simulink library "Library"  (R2017b)
settings: Solver=ode45  StartTime=0.0  StopTime=10.0  RelTol=1e-3  EnableMultiTasking=on
libraries: simulink x1
settings Model: Creator=Administrator  LastModifiedBy=ZhuDeShui
settings DataIOCC: LimitDataPoints=on  SaveFormat=Array
settings OptimizationCC: LifeSpan=inf
settings DebuggingCC: SolverPrmCheckMsg=warning  AllowSymbolicDim=off  SFUnexpectedBacktrackingDiag=warning  SFNoUnconditionalDefaultTransitionDiag=warning  SFExecutionAtInitializationDiag=none
settings HardwareCC: ProdBitPerPointer=32  ProdBitPerSizeT=32  ProdBitPerPtrDiffT=32  ProdLargestAtomicFloat=None  ProdIntDivRoundTo=Undefined  ProdEndianess=Unspecified  ProdWordSize=32  ProdHWDeviceType=32-bit Generic
settings ModelReferenceCC: PropagateSignalLabelsOutOfModel=off
settings CodeAppCC: StateflowObjectComments=on
settings GRTTargetCC: TargetLangStandard=C89/C90 (ANSI)  GeneratePreprocessorConditionals=Disable all
settings ConfigComp: CovMetricSettings=dw  CovHtmlReporting=on  CovSaveCumulativeToWorkspaceVar=on  CovSaveSingleToWorkspaceVar=on  CovExternalEMLEnable=off  CovSFcnEnable=off

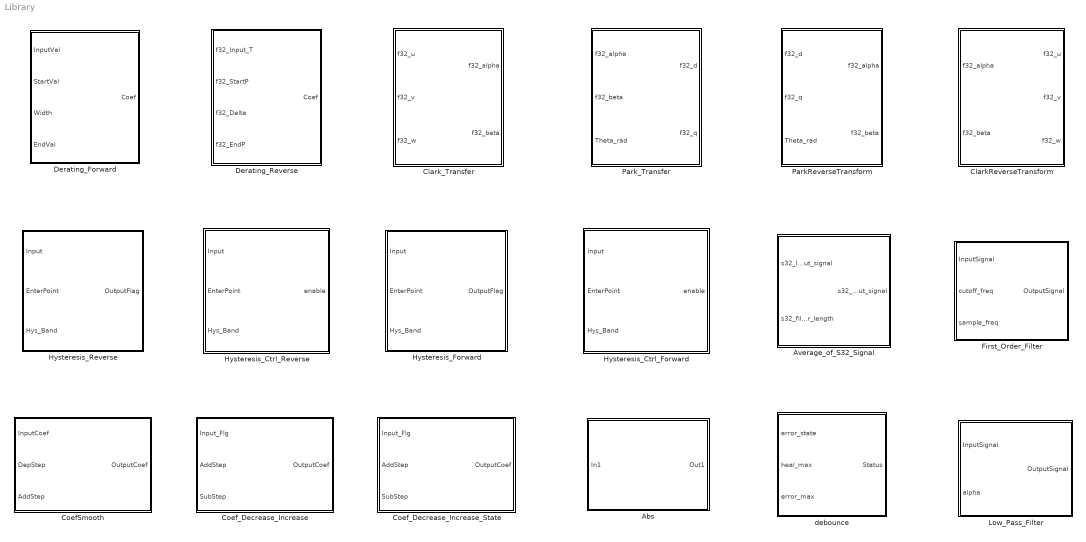
== system Library ==
  Abs : Subsystem  TreatAsAtomicUnit=on  RTWFcnName=Abs
      settings: RTWFcnNameOpts=User specified
  Average_of_S32_Signal : Subsystem  TreatAsAtomicUnit=on  RTWFcnName=Average_of_S32_Signal
      settings: RTWFcnNameOpts=User specified
  ClarkReverseTransform : Subsystem  TreatAsAtomicUnit=on  RTWFcnName=ClarkReverseTransform
      settings: RTWFcnNameOpts=User specified
  Clark_Transfer : Subsystem  TreatAsAtomicUnit=on  RTWFcnName=Clark_Transfer
      settings: RTWFcnNameOpts=User specified
  CoefSmooth : Subsystem  TreatAsAtomicUnit=on  RTWFcnName=CoefSmooth
      settings: RTWFcnNameOpts=User specified
  Coef_Decrease_Increase : Subsystem  TreatAsAtomicUnit=on  RTWFcnName=Coef_Decrease_Increase
      settings: RTWFcnNameOpts=User specified
  Coef_Decrease_Increase_State : Subsystem  TreatAsAtomicUnit=on  RTWFcnName=Coef_Decrease_Increase_State
      settings: RTWFcnNameOpts=User specified
  Derating_Forward : Subsystem  TreatAsAtomicUnit=on  RTWFcnName=Derating_Forward
      settings: RTWFcnNameOpts=User specified
  Derating_Reverse : Subsystem  TreatAsAtomicUnit=on  RTWFcnName=Derating_Reverse
      settings: RTWFcnNameOpts=User specified
  First_Order_Filter : Subsystem  TreatAsAtomicUnit=on  RTWFcnName=First_Order_Filter
      settings: RTWFcnNameOpts=User specified
  Hysteresis_Ctrl_Forward : Subsystem  TreatAsAtomicUnit=on  RTWFcnName=Hysteresis_Ctrl_Forward
      settings: RTWFcnNameOpts=User specified
  Hysteresis_Ctrl_Reverse : Subsystem  TreatAsAtomicUnit=on  RTWFcnName=Hysteresis_Ctrl_Reverse
      settings: RTWFcnNameOpts=User specified
  Hysteresis_Forward : Subsystem  TreatAsAtomicUnit=on  RTWFcnName=Hysteresis_Forward
      settings: RTWFcnNameOpts=User specified
  Hysteresis_Reverse : Subsystem  TreatAsAtomicUnit=on  RTWFcnName=Hysteresis_Reverse
      settings: RTWFcnNameOpts=User specified
  Low_Pass_Filter : Subsystem  TreatAsAtomicUnit=on  RTWFcnName=Low_Pass_Filter
      settings: RTWFcnNameOpts=User specified
  ParkReverseTransform : Subsystem  TreatAsAtomicUnit=on  RTWFcnName=ParkReverseTransform
      settings: RTWFcnNameOpts=User specified
  Park_Transfer : Subsystem  TreatAsAtomicUnit=on  RTWFcnName=Park_Transfer
      settings: RTWFcnNameOpts=User specified
  debounce : Subsystem  TreatAsAtomicUnit=on  RTWFcnName=debounce
      settings: RTWFcnNameOpts=User specified

== system Library/Abs ==
  In1 : Inport
  Compare To Zero : simulink/Logic and Bit Operations/Compare To Zero  relop=>=  OutDataTypeStr=boolean
  Gain : Gain  Gain=-1  OutDataTypeStr=single
  Switch : Switch  Criteria=u2 ~= 0
  Out1 : Outport
  wires:
  In1/1 -> Gain/1, Compare To Zero/1, Switch/1
  Compare To Zero/1 -> Switch/2
  Gain/1 -> Switch/3
  Switch/1 -> Out1/1

== system Library/Average_of_S32_Signal ==
  s32_Input_signal : Inport
  s32_filter_length : Inport  Port=2
  Chart : Stateflow chart  TreatAsAtomicUnit=on
  s32_Output_signal : Outport
  wires:
  Chart/1(s32_Output_signal) -> s32_Output_signal/1
  s32_filter_length/1 -> Chart/2(s32_filter_length)
  s32_Input_signal/1 -> Chart/1(s32_Input_signal)

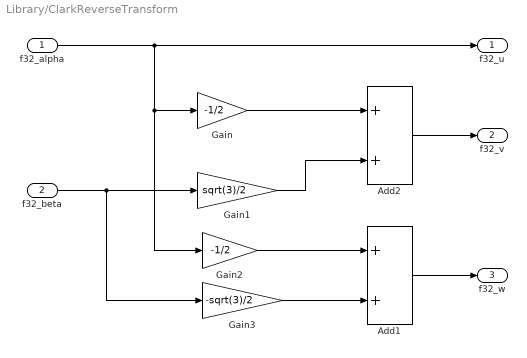
== system Library/ClarkReverseTransform ==
  f32_alpha : Inport  OutDataTypeStr=single
  f32_beta : Inport  Port=2  OutDataTypeStr=single
  Add1 : Sum  AccumDataTypeStr=single
  Add2 : Sum  OutDataTypeStr=single
  Gain : Gain  Gain=-1/2  OutDataTypeStr=single
  Gain1 : Gain  Gain=sqrt(3)/2  OutDataTypeStr=single
  Gain2 : Gain  Gain=-1/2  OutDataTypeStr=single
  Gain3 : Gain  Gain=-sqrt(3)/2  OutDataTypeStr=single
  f32_u : Outport  OutDataTypeStr=single
  f32_v : Outport  Port=2  OutDataTypeStr=single
  f32_w : Outport  Port=3  OutDataTypeStr=single
  wires:
  f32_alpha/1 -> Gain2/1, Gain/1, f32_u/1
  Gain/1 -> Add2/1
  Gain1/1 -> Add2/2
  f32_beta/1 -> Gain3/1, Gain1/1
  Gain2/1 -> Add1/1
  Gain3/1 -> Add1/2
  Add1/1 -> f32_w/1
  Add2/1 -> f32_v/1

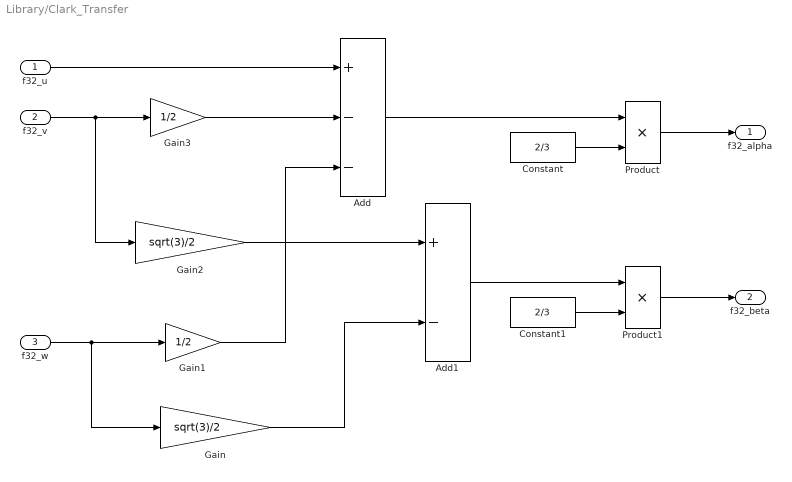
== system Library/Clark_Transfer ==
  f32_u : Inport
  f32_v : Inport  Port=2
  f32_w : Inport  Port=3
  Add : Sum  Inputs=+--
  Add1 : Sum  Inputs=+-
  Constant : Constant  Value=2/3  OutDataTypeStr=single
  Constant1 : Constant  Value=2/3  OutDataTypeStr=single
  Gain : Gain  Gain=sqrt(3)/2  OutDataTypeStr=single
  Gain1 : Gain  Gain=1/2  OutDataTypeStr=single
  Gain2 : Gain  Gain=sqrt(3)/2  OutDataTypeStr=single
  Gain3 : Gain  Gain=1/2  OutDataTypeStr=single
  Product : Product
  Product1 : Product
  f32_alpha : Outport
  f32_beta : Outport  Port=2
  wires:
  f32_w/1 -> Gain/1, Gain1/1
  Gain1/1 -> Add/3
  Gain/1 -> Add1/2
  f32_u/1 -> Add/1
  f32_v/1 -> Gain2/1, Gain3/1
  Gain3/1 -> Add/2
  Gain2/1 -> Add1/1
  Constant/1 -> Product/2
  Add/1 -> Product/1
  Product/1 -> f32_alpha/1
  Constant1/1 -> Product1/2
  Add1/1 -> Product1/1
  Product1/1 -> f32_beta/1

== system Library/CoefSmooth ==
  InputCoef : Inport
  DepStep : Inport  Port=2
  AddStep : Inport  Port=3
  Chart : Stateflow chart  TreatAsAtomicUnit=on
  OutputCoef : Outport
  wires:
  InputCoef/1 -> Chart/1(InputCoef)
  DepStep/1 -> Chart/2(DepStep)
  AddStep/1 -> Chart/3(AddStep)
  Chart/1(OutputCoef) -> OutputCoef/1

== system Library/Coef_Decrease_Increase ==
  Input_Flg : Inport
  AddStep : Inport  Port=2
  SubStep : Inport  Port=3
  Chart : Stateflow chart  TreatAsAtomicUnit=on
  OutputCoef : Outport
  wires:
  Input_Flg/1 -> Chart/1(Input_Flg)
  SubStep/1 -> Chart/3(SubStep)
  AddStep/1 -> Chart/2(AddStep)
  Chart/1(OutputCoef) -> OutputCoef/1

== system Library/Coef_Decrease_Increase_State ==
  Input_Flg : Inport
  AddStep : Inport  Port=2
  SubStep : Inport  Port=3
  Chart : Stateflow chart  TreatAsAtomicUnit=on
  OutputCoef : Outport
  wires:
  Chart/1(OutputCoef) -> OutputCoef/1
  AddStep/1 -> Chart/2(AddStep)
  SubStep/1 -> Chart/3(SubStep)
  Input_Flg/1 -> Chart/1(Input_Flg)

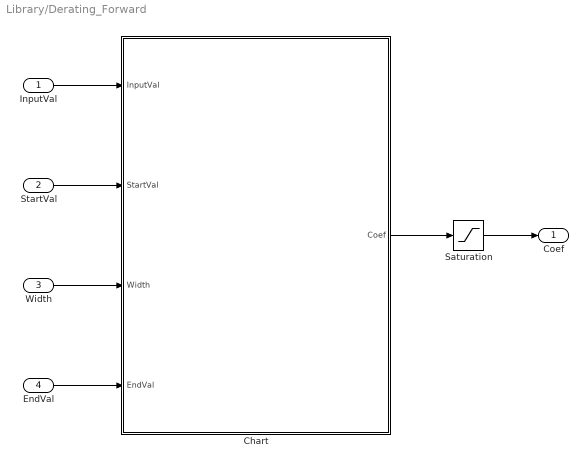
== system Library/Derating_Forward ==
  InputVal : Inport
  StartVal : Inport  Port=2
  Width : Inport  Port=3
  EndVal : Inport  Port=4
  Chart : Stateflow chart  TreatAsAtomicUnit=on
  Saturation : Saturate  UpperLimit=1  LowerLimit=0  OutDataTypeStr=single
  Coef : Outport
  wires:
  Saturation/1 -> Coef/1
  InputVal/1 -> Chart/1(InputVal)
  StartVal/1 -> Chart/2(StartVal)
  Width/1 -> Chart/3(Width)
  EndVal/1 -> Chart/4(EndVal)
  Chart/1(Coef) -> Saturation/1

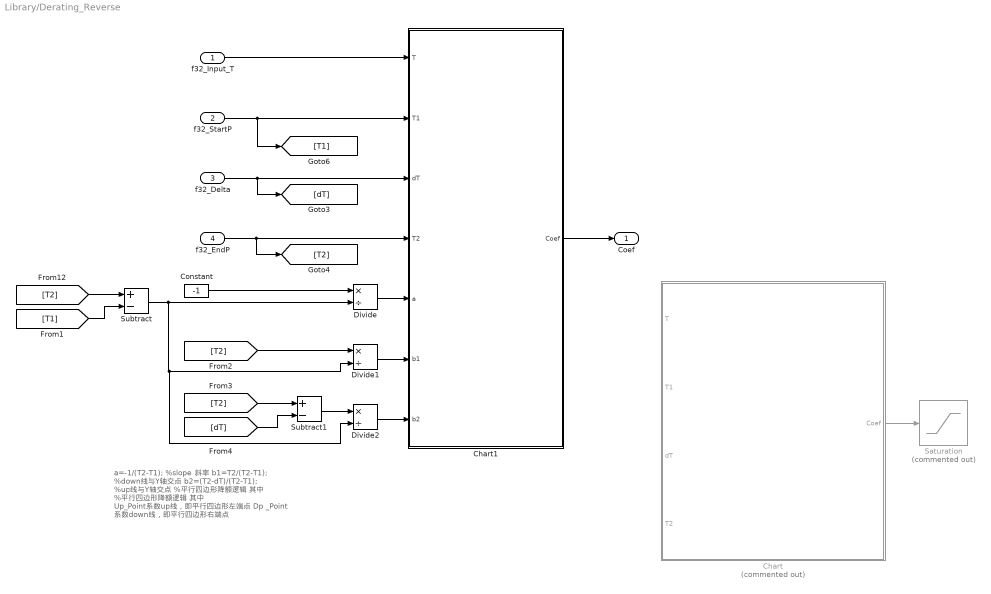
== system Library/Derating_Reverse ==
  note: a=-1/(T2-T1);                     %slope  斜率
      | b1=T2/(T2-T1);                  %down线与Y轴交点
      | b2=(T2-dT)/(T2-T1);          %up线与Y轴交点
      | %平行四边形降额逻辑
      | 其中
      | %平行四边形降额逻辑
      | 其中
      | Up_Point系数up线，即平行四边形左端点
      | Dp _Point 系数down线，即平行四边形右端点
  f32_Input_T : Inport
  f32_StartP : Inport  Port=2
  f32_Delta : Inport  Port=3
  f32_EndP : Inport  Port=4
  Chart : Stateflow chart  Commented=on  TreatAsAtomicUnit=on
  Chart1 : Stateflow chart  TreatAsAtomicUnit=on
  Constant : Constant  Value=-1  OutDataTypeStr=single
  Divide : Product  Inputs=*/
  Divide1 : Product  Inputs=*/
  Divide2 : Product  Inputs=*/
  Saturation : Saturate  Commented=on  UpperLimit=1  LowerLimit=0  OutDataTypeStr=single
  Subtract : Sum  Inputs=+-
  Subtract1 : Sum  Inputs=+-
  Coef : Outport
  wires:
  Chart/1(Coef) -> Saturation/1
  f32_StartP/1 -> [T1], Chart1/2(T1)
  f32_Input_T/1 -> Chart1/1(T)
  f32_Delta/1 -> [dT], Chart1/3(dT)
  f32_EndP/1 -> [T2], Chart1/4(T2)
  Chart1/1(Coef) -> Coef/1
  Divide/1 -> Chart1/5(a)
  Constant/1 -> Divide/1
  Subtract/1 -> Divide2/2, Divide1/2, Divide/2
  [T2] -> Subtract/1
  [T1] -> Subtract/2
  Divide1/1 -> Chart1/6(b1)
  [T2] -> Divide1/1
  Divide2/1 -> Chart1/7(b2)
  Subtract1/1 -> Divide2/1
  [T2] -> Subtract1/1
  [dT] -> Subtract1/2

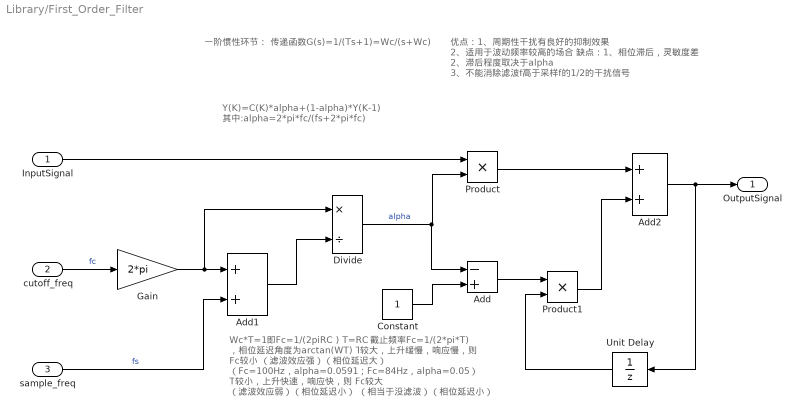
== system Library/First_Order_Filter ==
  note: 一阶惯性环节：
      | 传递函数G(s)=1/(Ts+1)=Wc/(s+Wc)
  note: 优点：1、周期性干扰有良好的抑制效果
      | 2、适用于波动频率较高的场合
      | 缺点：1、相位滞后，灵敏度差
      | 2、滞后程度取决于alpha
      | 3、不能消除滤波f高于采样f的1/2的干扰信号
  note: Wc*T=1即Fc=1/(2piRC ) T=RC
      | 截止频率Fc=1/(2*pi*T) ，相位延迟角度为arctan(WT)
      | T较大，上升缓慢，响应慢，则 Fc较小
      | （滤波效应强）（相位延迟大）
      | （Fc=100Hz，alpha=0.0591；Fc=84Hz，alpha=0.05）
      | T较小，上升快速，响应快，则 Fc较大
      | （滤波效应弱）（相位延迟小）
      | （相当于没滤波）（相位延迟小）
  note: Y(K)=C(K)*alpha+(1-alpha)*Y(K-1)
      |
      | 其中:alpha=2*pi*fc/(fs+2*pi*fc)
  InputSignal : Inport  OutDataTypeStr=single
  cutoff_freq : Inport  Port=2  OutDataTypeStr=single
  sample_freq : Inport  Port=3  OutDataTypeStr=single
  Add : Sum  Inputs=-+  OutDataTypeStr=single
  Add1 : Sum  OutDataTypeStr=single
  Add2 : Sum  OutDataTypeStr=single
  Constant : Constant  OutDataTypeStr=single
  Divide : Product  Inputs=*/  OutDataTypeStr=single
  Gain : Gain  Gain=2*pi  ParamDataTypeStr=single  OutDataTypeStr=single
  Product : Product  OutDataTypeStr=single
  Product1 : Product  OutDataTypeStr=single
  Unit Delay : UnitDelay  SampleTime=-1
  OutputSignal : Outport
  wires:
  cutoff_freq/1 -> Gain/1  "fc"
  Gain/1 -> Divide/1, Add1/1
  sample_freq/1 -> Add1/2  "fs"
  InputSignal/1 -> Product/1
  Add1/1 -> Divide/2
  Divide/1 -> Add/1, Product/2  "alpha"
  Constant/1 -> Add/2
  Add/1 -> Product1/1
  Product1/1 -> Add2/2
  Product/1 -> Add2/1
  Add2/1 -> Unit Delay/1, OutputSignal/1
  Unit Delay/1 -> Product1/2

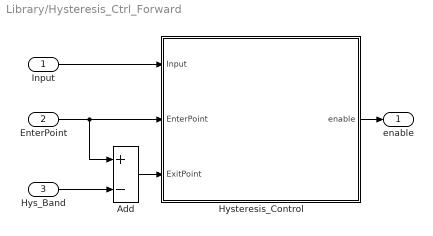
== system Library/Hysteresis_Ctrl_Forward ==
  Input : Inport
  EnterPoint : Inport  Port=2
  Hys_Band : Inport  Port=3
  Add : Sum  Inputs=+-
  Hysteresis_Control : Stateflow chart  TreatAsAtomicUnit=on
  enable : Outport  OutDataTypeStr=boolean
  wires:
  Hys_Band/1 -> Add/2
  Add/1 -> Hysteresis_Control/3(ExitPoint)
  Hysteresis_Control/1(enable) -> enable/1
  Input/1 -> Hysteresis_Control/1(Input)
  EnterPoint/1 -> Add/1, Hysteresis_Control/2(EnterPoint)

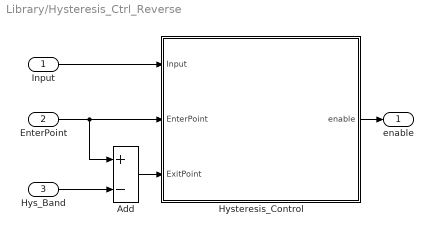
== system Library/Hysteresis_Ctrl_Reverse ==
  Input : Inport
  EnterPoint : Inport  Port=2
  Hys_Band : Inport  Port=3
  Add : Sum  Inputs=+-
  Hysteresis_Control : Stateflow chart  TreatAsAtomicUnit=on
  enable : Outport  OutDataTypeStr=boolean
  wires:
  Hys_Band/1 -> Add/2
  Add/1 -> Hysteresis_Control/3(ExitPoint)
  Hysteresis_Control/1(enable) -> enable/1
  Input/1 -> Hysteresis_Control/1(Input)
  EnterPoint/1 -> Add/1, Hysteresis_Control/2(EnterPoint)

== system Library/Hysteresis_Forward ==
  Input : Inport
  EnterPoint : Inport  Port=2
  Hys_Band : Inport  Port=3
  Add1 : Sum  Inputs=+-
  Hysteresis_Ctrl : Stateflow chart  TreatAsAtomicUnit=on
  OutputFlag : Outport
  wires:
  Hys_Band/1 -> Add1/2
  Input/1 -> Hysteresis_Ctrl/1(InputSignal)
  EnterPoint/1 -> Hysteresis_Ctrl/2(EnterPoint), Add1/1
  Add1/1 -> Hysteresis_Ctrl/3(ExitPoint)
  Hysteresis_Ctrl/1(OutputFlag) -> OutputFlag/1

== system Library/Hysteresis_Reverse ==
  Input : Inport
  EnterPoint : Inport  Port=2
  Hys_Band : Inport  Port=3
  Add1 : Sum  Inputs=+-
  Hysteresis_Ctrl : Stateflow chart  TreatAsAtomicUnit=on
  OutputFlag : Outport
  wires:
  Hysteresis_Ctrl/1(OutputFlag) -> OutputFlag/1
  Add1/1 -> Hysteresis_Ctrl/3(ExitPoint)
  EnterPoint/1 -> Add1/1, Hysteresis_Ctrl/2(EnterPoint)
  Input/1 -> Hysteresis_Ctrl/1(InputSignal)
  Hys_Band/1 -> Add1/2

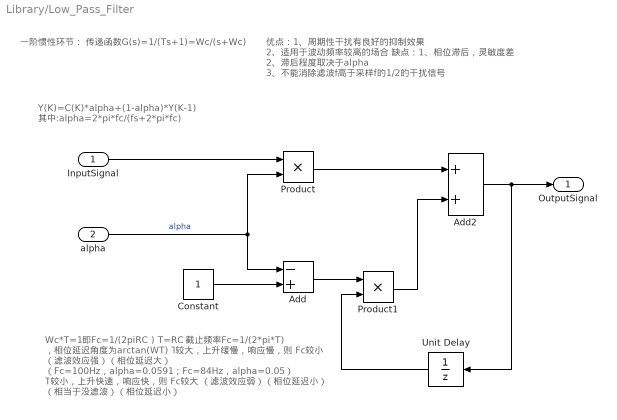
== system Library/Low_Pass_Filter ==
  note: Wc*T=1即Fc=1/(2piRC ) T=RC
      | 截止频率Fc=1/(2*pi*T) ，相位延迟角度为arctan(WT)
      | T较大，上升缓慢，响应慢，则 Fc较小
      | （滤波效应强）（相位延迟大）
      | （Fc=100Hz，alpha=0.0591；Fc=84Hz，alpha=0.05）
      | T较小，上升快速，响应快，则 Fc较大
      | （滤波效应弱）（相位延迟小）
      | （相当于没滤波）（相位延迟小）
  note: 优点：1、周期性干扰有良好的抑制效果
      | 2、适用于波动频率较高的场合
      | 缺点：1、相位滞后，灵敏度差
      | 2、滞后程度取决于alpha
      | 3、不能消除滤波f高于采样f的1/2的干扰信号
  note: 一阶惯性环节：
      | 传递函数G(s)=1/(Ts+1)=Wc/(s+Wc)
  note: Y(K)=C(K)*alpha+(1-alpha)*Y(K-1)
      |
      | 其中:alpha=2*pi*fc/(fs+2*pi*fc)
  InputSignal : Inport  OutDataTypeStr=single
  alpha : Inport  Port=2  OutDataTypeStr=single
  Add : Sum  Inputs=-+  OutDataTypeStr=single
  Add2 : Sum  OutDataTypeStr=single
  Constant : Constant  OutDataTypeStr=single
  Product : Product  OutDataTypeStr=single
  Product1 : Product  OutDataTypeStr=single
  Unit Delay : UnitDelay  SampleTime=-1
  OutputSignal : Outport
  wires:
  Add/1 -> Product1/1
  Product1/1 -> Add2/2
  Add2/1 -> Unit Delay/1, OutputSignal/1
  alpha/1 -> Product/2, Add/1  "alpha"
  Constant/1 -> Add/2
  Product/1 -> Add2/1
  Unit Delay/1 -> Product1/2
  InputSignal/1 -> Product/1

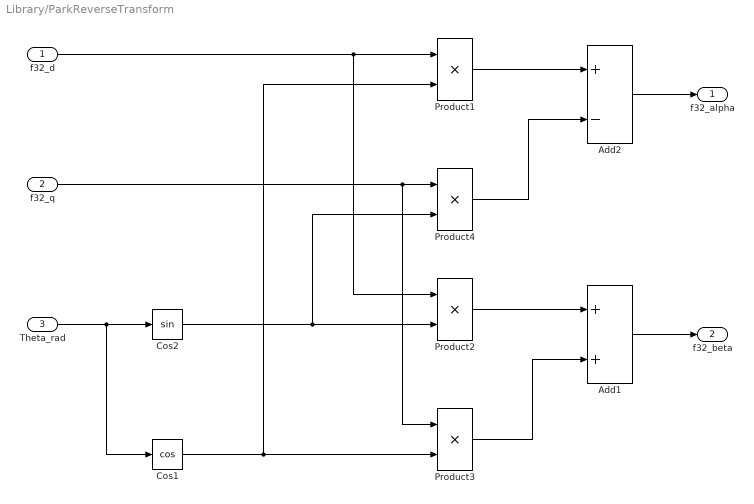
== system Library/ParkReverseTransform ==
  f32_d : Inport  OutDataTypeStr=single
  f32_q : Inport  Port=2  OutDataTypeStr=single
  Theta_rad : Inport  Port=3  OutDataTypeStr=single
  Add1 : Sum  OutDataTypeStr=single
  Add2 : Sum  Inputs=+-  OutDataTypeStr=single
  Cos1 : Trigonometry  Operator=cos
  Cos2 : Trigonometry
  Product{1..4} (4 alike) : Product  OutDataTypeStr=single
  f32_alpha : Outport  OutDataTypeStr=single
  f32_beta : Outport  Port=2  OutDataTypeStr=single
  wires:
  Theta_rad/1 -> Cos1/1, Cos2/1
  Add2/1 -> f32_alpha/1
  Add1/1 -> f32_beta/1
  Product1/1 -> Add2/1
  Product4/1 -> Add2/2
  Product2/1 -> Add1/1
  Product3/1 -> Add1/2
  f32_d/1 -> Product2/1, Product1/1
  Cos1/1 -> Product3/2, Product1/2
  f32_q/1 -> Product3/1, Product4/1
  Cos2/1 -> Product4/2, Product2/2

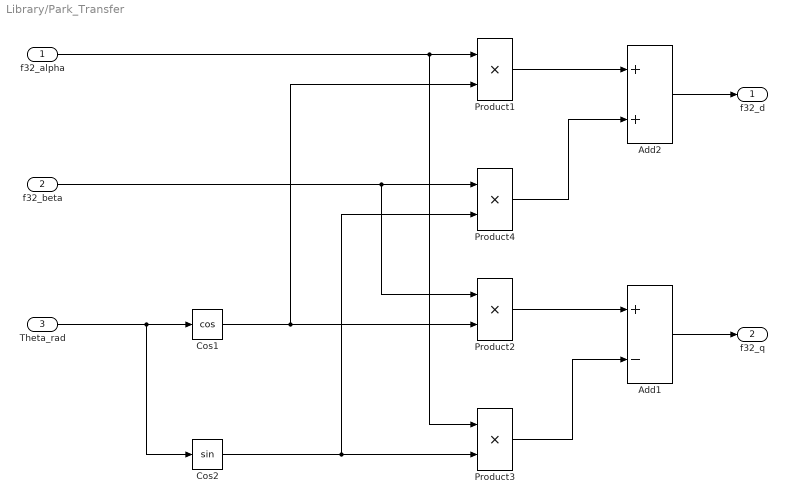
== system Library/Park_Transfer ==
  f32_alpha : Inport
  f32_beta : Inport  Port=2
  Theta_rad : Inport  Port=3  OutDataTypeStr=single
  Add1 : Sum  Inputs=+-
  Add2 : Sum
  Cos1 : Trigonometry  Operator=cos
  Cos2 : Trigonometry
  Product{1..4} (4 alike) : Product
  f32_d : Outport
  f32_q : Outport  Port=2
  wires:
  Theta_rad/1 -> Cos1/1, Cos2/1
  Add2/1 -> f32_d/1
  Add1/1 -> f32_q/1
  f32_alpha/1 -> Product3/1, Product1/1
  f32_beta/1 -> Product2/1, Product4/1
  Cos1/1 -> Product2/2, Product1/2
  Cos2/1 -> Product4/2, Product3/2
  Product1/1 -> Add2/1
  Product4/1 -> Add2/2
  Product2/1 -> Add1/1
  Product3/1 -> Add1/2

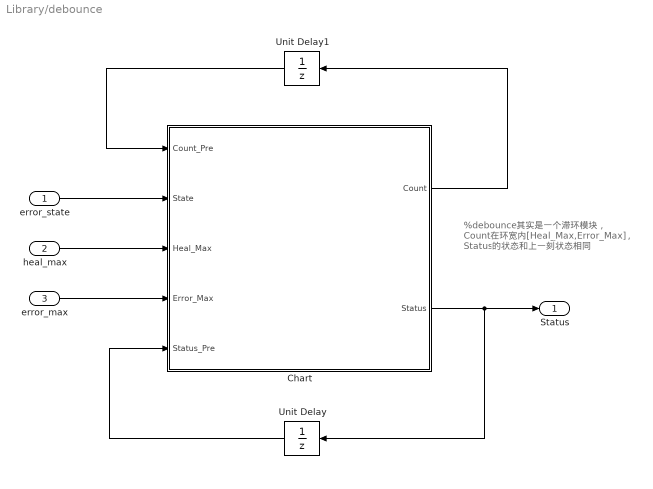
== system Library/debounce ==
  note: %debounce其实是一个滞环模块，
      | Count在环宽内[Heal_Max,Error_Max]，
      | Status的状态和上一刻状态相同
  error_state : Inport  OutDataTypeStr=boolean
  heal_max : Inport  Port=2  OutDataTypeStr=int16
  error_max : Inport  Port=3  OutDataTypeStr=int16
  Chart : Stateflow chart  TreatAsAtomicUnit=on
  Unit Delay : UnitDelay  SampleTime=-1
  Unit Delay1 : UnitDelay  SampleTime=-1
  Status : Outport
  wires:
  Chart/2(Status) -> Unit Delay/1, Status/1
  heal_max/1 -> Chart/3(Heal_Max)
  error_state/1 -> Chart/2(State)
  error_max/1 -> Chart/4(Error_Max)
  Chart/1(Count) -> Unit Delay1/1
  Unit Delay1/1 -> Chart/1(Count_Pre)
  Unit Delay/1 -> Chart/5(Status_Pre)

== stateflow chart Library/debounce/Chart ==
  note: %故障来了
  note: %故障发生前，计算器为负值
  note: %没有故障
  note: %计算器由负值立即置2
  note: %Count一次减1
  note: %Count一次加2
  note: %Count小于下限  或者  上个Status为0且Count处于[Heal_Max,Error_Max]，输出的Status为0
      | %在滞环内，State的输出不变，和上一刻的状态State一样
  (default) -> (junction 8)
  (junction 8) -> (junction 10) [order 1] : [State==1]
  (junction 8) -> (junction 12) [order 2]
  (junction 10) -> (junction 22)
  (junction 22) -> (junction 30) [order 1] : [Count_Pre<=0]
  (junction 22) -> (junction 24) [order 2]
  (junction 30) -> (junction 36) : {
      | Count=2;
      | }
  (junction 12) -> (junction 14) [order 1] : [Count_Pre<=Heal_Max]
  (junction 12) -> (junction 17) [order 2] : {
      | Count=Count_Pre-1;
      | }
  (junction 14) -> (junction 16) : {
      | Count=Heal_Max;
      | }
  (junction 24) -> (junction 32) [order 1] : [Count_Pre>=Error_Max]
  (junction 24) -> (junction 26) [order 2] : {
      | Count=Count_Pre+2;
      | }
  (junction 32) -> (junction 34) : {
      | Count=Error_Max;
      | }
  (junction 16) -> (junction 17)
  (junction 17) -> (junction 40)
  (junction 34) -> (junction 26)
  (junction 36) -> (junction 34)
  (junction 26) -> (junction 28)
  (junction 28) -> (junction 40)
  (junction 40) -> (junction 43)
  (junction 43) -> (junction 45) [order 1] : [(Count<=Heal_Max)||((Status_Pre<=0)&&(Heal_Max<Count)&&(Count<Error_Max))]
  (junction 43) -> (junction 47) [order 2] : {
      | Status=1;
      | }
  (junction 45) -> (junction 49) : {
      | Status=0;
      | }
  (junction 49) -> (junction 47)
  (junction 47) -> (junction 52)
  data: Count_Pre input int16; State input boolean; Heal_Max input int16; Error_Max input int16; Status_Pre input boolean; Count output int16; Status output boolean

== stateflow chart Library/Hysteresis_Forward/Hysteresis_Ctrl ==
  note: InputSignal在[ExitPoint,EnterPoint]
      | 没有状态的跳转，即保持原来的状态输出
  state On
    en:
    OutputFlag=1;
  state Off
    en:
    OutputFlag=0;
  (default) -> Off
  Off -> On : [InputSignal>=EnterPoint]
  On -> Off : [InputSignal<=ExitPoint]
  data: InputSignal input single; OutputFlag output boolean; EnterPoint input single; ExitPoint input single

== stateflow chart Library/Derating_Reverse/Chart ==
  note: %平行四边形降额逻辑
  note: 其中
      | Up_Point系数up线，即平行四边形左端点
      | Dp _Point 系数down线，即平行四边形右端点
  note: 平行四边形右边为down线：表达式aT+b1
      | 平行四边形左边为up线表达式为：aT+b2
  state Initial
    note: [T1-dT,T1]
    note: 温度大于T1
    note: Up_point、Down_point之间，即平行四边形横边是降额系数不变
        | Up_point、Down_point、Current_Coef是局部变量
    (default) -> (junction 8)
    (junction 8) -> (junction 9) [order 1] : [T<T1-dT]
    (junction 9) -> (junction 12) : {
        | Coef=1;
        | }
    (junction 8) -> (junction 15) [order 2]
    (junction 15) -> (junction 17) [order 1] : [T<T1]
    (junction 15) -> (junction 20) [order 2] : {
        | Coef=a*T+b1;
        | Current_Coef=a*T+b1;
        | Up_point=T-dT;
        | Down_point=T;
        | }
    (junction 17) -> (junction 19) : {
        | Coef=1;
        | Current_Coef=1;
        | Up_point=T1-dT;
        | Down_point=T1;
        | }
    (junction 19) -> (junction 20)
    (junction 12) -> (junction 19)
    (junction 20) -> (junction 26)
  state HoldOn
    (default) -> (junction 51)
    HoldOn -> (junction 51) [order 1]
    (junction 51) -> (junction 53) : {
        | Coef=1;
        | Current_Coef=1;
        | Up_point=T1-dT;
        | Down_point=T1;
        | }
  state Judge
    note: 温度继续上升
    note: up点和down点之间，系数
        | 不变，继承上次的值
    note: 小于up点
    (default) -> (junction 87)
    Judge -> (junction 87) [order 1]
    (junction 87) -> (junction 90) [order 1] : [(T>=Down_point)&&(T<=T2)]
    (junction 87) -> (junction 92) [order 2]
    (junction 90) -> (junction 101) : {
        | Coef=a*T+b1;
        | Current_Coef=a*T+b1;
        | Up_point=T-dT;
        | Down_point=T;
        | }
    (junction 92) -> (junction 94) [order 1] : [T>Up_point]
    (junction 92) -> (junction 96) [order 2] : {
        | Coef=a*T+b2;
        | Current_Coef=a*T+b2;
        | Up_point=T;
        | Down_point=T+dT;
        | }
    (junction 94) -> (junction 98) : {
        | Coef=Current_Coef;
        | }
    (junction 98) -> (junction 96)
    (junction 101) -> (junction 98)
    (junction 96) -> (junction 138)
  (default) -> Initial : {
      | a=-1/(T2-T1);                     %slope  斜率
      | b1=T2/(T2-T1);                  %down线与Y轴交点
      | b2=(T2-dT)/(T2-T1);          %up线与Y轴交点
      | }
  Initial -> Judge [order 2] : [T>=T1-dT]
  Initial -> HoldOn [order 1]
  Judge -> HoldOn [order 1] : [T<T1-dT]
  HoldOn -> Judge [order 1] : [T>=T1-dT]
  data: T input single; Coef output single; Up_point local single; Down_point local single; Current_Coef local single; a local single; b1 local single; b2 local single; T1 input single; dT input single; T2 input single

== stateflow chart Library/Derating_Reverse/Chart1 ==
  state Initial
    (default) -> (junction 8)
    (junction 8) -> (junction 9) [order 1] : [T>T2]
    (junction 9) -> (junction 12) : {
        | Coef=0;
        | %Current_Coef=1;
        | Up_point=T2-dT;
        | Down_point=T2;
        | }
    (junction 8) -> (junction 15) [order 2]
    (junction 15) -> (junction 17) [order 1] : [T<T1]
    (junction 15) -> (junction 20) [order 2] : {
        | Coef=a*T+b1;
        | %Current_Coef=a*T+b1;
        | Up_point=T-dT;
        | Down_point=T;
        | }
    (junction 17) -> (junction 19) : {
        | Coef=1;
        | %Current_Coef=1;
        | Up_point=T1-dT;
        | Down_point=T1;
        | }
    (junction 19) -> (junction 20)
    (junction 12) -> (junction 19)
    (junction 20) -> (junction 26)
  state Judge
    (default) -> (junction 87)
    Judge -> (junction 87)
    (junction 87) -> (junction 90) [order 1] : [T<T1-dT]
    (junction 87) -> (junction 141) [order 2]
    (junction 90) -> (junction 101) : {
        | Coef=1;
        | %Current_Coef=1;
        | Up_point=T1-dT;
        | Down_point=T1;
        | }
    (junction 141) -> (junction 143) [order 1] : [T>T2]
    (junction 141) -> (junction 92) [order 2]
    (junction 143) -> (junction 150) : {
        | Coef=0;
        | %Current_Coef=a*T+b1;
        | Up_point=T2-dT;
        | Down_point=T2;
        | }
    (junction 92) -> (junction 94) [order 1] : [T>=Down_point]
    (junction 92) -> (junction 146) [order 2]
    (junction 94) -> (junction 98) : {
        | Coef=a*T+b1;
        | %Current_Coef=a*T+b1;
        | Up_point=T-dT;
        | Down_point=T;
        | }
    (junction 146) -> (junction 147) [order 1] : [T>Up_point]
    (junction 146) -> (junction 96) [order 2] : {
        | Coef=a*T+b2;
        | %Current_Coef=a*T+b2;
        | Up_point=T;
        | Down_point=T+dT;
        | }
    (junction 147) -> (junction 152) : {
        | %Coef=Current_Coef;
        | }
    (junction 152) -> (junction 96)
    (junction 98) -> (junction 152)
    (junction 150) -> (junction 98)
    (junction 101) -> (junction 150)
    (junction 96) -> (junction 138)
  (default) -> Initial
  Initial -> Judge : [1]
  data: T input single; T1 input single; dT input single; T2 input single; Coef output single; Up_point local single; Down_point local single; Current_Coef local single; a input single; b1 input single; b2 input single

== stateflow chart Library/CoefSmooth/Chart ==
  state y=funmax(m,n) [function]
    (default) -> (junction 3)
    (junction 3) -> (junction 11) [order 1] : [m>n]
    (junction 3) -> (junction 1) [order 2] : {
        | y=n;
        | }
    (junction 11) -> (junction 13) : {
        | y=m;
        | }
    (junction 13) -> (junction 1)
    (junction 1) -> (junction 15)
  note: 编写图像函数，函数名字
      | 不要和matlab函数重名
  state y=funmin(m,n) [function]
    (default) -> (junction 24)
    (junction 24) -> (junction 6) [order 1] : [m>n]
    (junction 24) -> (junction 23) [order 2] : {
        | y=m;
        | }
    (junction 6) -> (junction 2) : {
        | y=n;
        | }
    (junction 2) -> (junction 23)
    (junction 23) -> (junction 4)
  (default) -> (junction 40)
  (junction 40) -> (junction 41) [order 1] : [InputCoef>OutputCoef]
  (junction 40) -> (junction 38) [order 2] : {
      | OutputCoef=OutputCoef-DepStep;
      | OutputCoef=funmax(OutputCoef,InputCoef);
      | }
  (junction 41) -> (junction 42) : {
      | OutputCoef=OutputCoef+AddStep;
      | OutputCoef=funmin(OutputCoef,InputCoef);
      | }
  (junction 42) -> (junction 38)
  (junction 38) -> (junction 33)
  data: m function_input single; n function_input single; y function_output single; m function_input single; n function_input single; y function_output single; InputCoef input single; DepStep input single; OutputCoef output single =1; AddStep input single

== stateflow chart Library/Hysteresis_Ctrl_Forward/Hysteresis_Control ==
  note: Input属于[ExitPoint,
      | EnterPoint]，输出的
      | 标志位不进行赋值处理
  (default) -> (junction 6)
  (junction 6) -> (junction 7) [order 1] : [Input>=EnterPoint]
  (junction 6) -> (junction 11) [order 2]
  (junction 7) -> (junction 9) : {
      | enable=1;
      | }
  (junction 11) -> (junction 13) [order 1] : [Input<=ExitPoint]
  (junction 11) -> (junction 15) [order 2]
  (junction 13) -> (junction 16) : {
      | enable=0;
      | }
  (junction 16) -> (junction 15)
  (junction 9) -> (junction 16)
  (junction 15) -> (junction 21)
  data: Input input single; EnterPoint input single; ExitPoint input single; enable output boolean

== stateflow chart Library/Derating_Forward/Chart ==
  (default) -> (junction 11)
  (junction 11) -> (junction 14) [order 1] : [FirstFlag==0]
  (junction 11) -> (junction 13) [order 2]
  (junction 14) -> (junction 15) : {
      | DownVal=StartVal;
      | UpVal=StartVal+Width;
      | FirstFlag=1;
      | }
  (junction 15) -> (junction 13)
  (junction 13) -> (junction 20)
  (junction 20) -> (junction 22) [order 1] : [InputVal<=EndVal]
  (junction 20) -> (junction 26) [order 2]
  (junction 22) -> (junction 23) : {
      | DownVal=EndVal;
      | UpVal=EndVal+Width;
      | }
  (junction 26) -> (junction 27) [order 1] : [InputVal>=(StartVal+Width)]
  (junction 26) -> (junction 29) [order 2]
  (junction 27) -> (junction 28) : {
      | UpVal=StartVal+Width;
      | DownVal=StartVal;
      | }
  (junction 29) -> (junction 30) [order 1] : [InputVal>UpVal]
  (junction 29) -> (junction 45) [order 2]
  (junction 30) -> (junction 31) : {
      | UpVal=InputVal;
      | DownVal=UpVal-Width;
      | }
  (junction 45) -> (junction 46) [order 1] : [InputVal<DownVal]
  (junction 45) -> (junction 37) [order 2]
  (junction 46) -> (junction 44) : {
      | DownVal=InputVal;
      | UpVal=DownVal+Width;
      | }
  (junction 44) -> (junction 37)
  (junction 31) -> (junction 44)
  (junction 28) -> (junction 31)
  (junction 23) -> (junction 28)
  (junction 37) -> (junction 54) : {
      | Coef=(DownVal-EndVal)/(StartVal-EndVal);
      | }
  (junction 54) -> (junction 56)
  data: InputVal input single; StartVal input single; Width input single; Coef output single =1; DownVal local single size=1; EndVal input single; UpVal local single size=1; FirstFlag local boolean size=1 =0

== stateflow chart Library/Hysteresis_Ctrl_Reverse/Hysteresis_Control ==
  note: Input属于[ExitPoint,
      | EnterPoint]，输出的
      | 标志位不进行赋值处理
  (default) -> (junction 6)
  (junction 6) -> (junction 7) [order 1] : [Input>=EnterPoint]
  (junction 6) -> (junction 11) [order 2]
  (junction 7) -> (junction 9) : {
      | enable=0;
      | }
  (junction 11) -> (junction 13) [order 1] : [Input<=ExitPoint]
  (junction 11) -> (junction 15) [order 2]
  (junction 13) -> (junction 16) : {
      | enable=1;
      | }
  (junction 16) -> (junction 15)
  (junction 9) -> (junction 16)
  (junction 15) -> (junction 21)
  data: Input input single; EnterPoint input single; ExitPoint input single; enable output boolean

== stateflow chart Library/Hysteresis_Reverse/Hysteresis_Ctrl ==
  note: InputSignal在[ExitPoint,EnterPoint]
      | 没有状态的跳转，即保持原来的状态输出
  state On
    en:
    OutputFlag=0;
  state Off
    en:
    OutputFlag=1;
  (default) -> Off
  Off -> On : [InputSignal>=EnterPoint]
  On -> Off : [InputSignal<=ExitPoint]
  data: InputSignal input single; OutputFlag output boolean; EnterPoint input single; ExitPoint input single

== stateflow chart Library/Coef_Decrease_Increase_State/Chart ==
  state Normal
    en:
    OutputCoef=1;
    Coef_Local=OutputCoef;
    du:
    OutputCoef=1;
    Coef_Local=OutputCoef;
  state Coef_Increase
    (default) -> (junction 124) : {
        | OutputCoef=Coef_Local;
        | }
    Coef_Increase -> (junction 124) [order 1]
    (junction 124) -> (junction 125) : {
        | OutputCoef=OutputCoef+AddStep;
        | Coef_Local=OutputCoef;
        | }
    (junction 125) -> (junction 134) [order 1] : [OutputCoef>=1]
    (junction 125) -> (junction 123) [order 2]
    (junction 134) -> (junction 130) : {
        | OutputCoef=1;
        | Coef_Local=1;
        | }
    (junction 130) -> (junction 123)
    (junction 123) -> (junction 126)
  state Coef_Decrease
    (default) -> (junction 62) : {
        | OutputCoef=Coef_Local;
        | }
    Coef_Decrease -> (junction 62) [order 1]
    (junction 62) -> (junction 66) : {
        | OutputCoef=OutputCoef-SubStep;
        | Coef_Local=OutputCoef;
        | }
    (junction 66) -> (junction 67) [order 1] : [OutputCoef<=0]
    (junction 66) -> (junction 70) [order 2]
    (junction 67) -> (junction 71) : {
        | OutputCoef=0;
        | Coef_Local=0;
        | }
    (junction 71) -> (junction 70)
    (junction 70) -> (junction 72)
  note: 有故障时候，Coef线性降到0
  note: 故障消失后，Coef
      | 线性增大到1
  note: 继承Coef，相当于加一个local变量
  (default) -> Normal
  Coef_Increase -> Normal [order 1] : [OutputCoef==1]
  Normal -> Coef_Decrease : [Input_Flg>=1]
  Coef_Decrease -> Coef_Increase [order 1] : [Input_Flg<=0]
  Coef_Increase -> Coef_Decrease [order 2] : [Input_Flg>=1]
  data: Input_Flg input boolean; AddStep input single; SubStep input single; OutputCoef output single; Coef_Local local single

== stateflow chart Library/Coef_Decrease_Increase/Chart ==
  state y=funmax(m,n) [function]
    (default) -> (junction 3)
    (junction 3) -> (junction 11) [order 1] : [m>n]
    (junction 3) -> (junction 1) [order 2] : {
        | y=n;
        | }
    (junction 11) -> (junction 13) : {
        | y=m;
        | }
    (junction 13) -> (junction 1)
    (junction 1) -> (junction 15)
  note: 当Flg=1，Coef_Local由初值1开始降，
      | 当降到0时候，保持为0
  note: 当Flg=0，
      | Coef_Local开始
      | 恢复，趋近于1，
      | 超过1后，保持为1
  note: 编写图像函数，函数名字
      | 不要和matlab函数重名
  state y=funmin(m,n) [function]
    (default) -> (junction 24)
    (junction 24) -> (junction 6) [order 1] : [m>n]
    (junction 24) -> (junction 23) [order 2] : {
        | y=m;
        | }
    (junction 6) -> (junction 2) : {
        | y=n;
        | }
    (junction 2) -> (junction 23)
    (junction 23) -> (junction 4)
  note: Coef_Local局部变量初值为1
  (default) -> (junction 40)
  (junction 40) -> (junction 41) [order 1] : [Input_Flg==1]
  (junction 40) -> (junction 38) [order 2] : {
      | Coef_Local=Coef_Local+AddStep;
      | Coef_Local=funmin(Coef_Local,1);
      | }
  (junction 41) -> (junction 42) : {
      | Coef_Local=Coef_Local-SubStep;
      | Coef_Local=funmax(Coef_Local,0);
      | }
  (junction 42) -> (junction 38)
  (junction 38) -> (junction 33) : {
      | OutputCoef=Coef_Local;
      | }
  data: m function_input single; n function_input single; y function_output single; m function_input single; n function_input single; y function_output single; Input_Flg input boolean; AddStep input single; SubStep input single; OutputCoef output single; Coef_Local local single =1

== stateflow chart Library/Average_of_S32_Signal/Chart ==
  note: f32_Buff[i]是？定义size为2000？
  (default) -> (junction 8) : {
      | s32_Sum=s32_Sum-s32_Buff[i]+s32_Input_signal;
      | s32_Output_signal=s32_Sum/s32_filter_length;
      | s32_Buff[i]=s32_Input_signal;
      | i=i+1;
      | }
  (junction 8) -> (junction 9) [order 1] : [i>=s32_filter_length]
  (junction 8) -> (junction 10) [order 2]
  (junction 9) -> (junction 11) : {
      | i=0;
      | }
  (junction 11) -> (junction 10)
  (junction 10) -> (junction 17)
  data: s32_Input_signal input int32; s32_filter_length input int32; s32_Output_signal output int32; i local int32; s32_Sum local int32; s32_Buff local int32 size=2000
